simulink model "martalg1"  (Simulink 6.1)
settings: Solver=ode45  StartTime=0.0  StopTime=10.0  RelTol=1e-3
settings Model: Creator=pmosterm  LastModifiedBy=mshakeri  ExtModeAutoUpdateStatusClock=off  StrictBusMsg=ErrorLevel1
settings DataIOCC: SaveFormat=StructureWithTime  SignalLoggingName=logsOut
settings OptimizationCC: InlineParams=on  OptimizeModelRefInitCode=on  LifeSpan=1
settings ModelReferenceCC: ModelReferenceMinAlgLoopOccurrences=on
settings RTWCC: SystemTargetFile=ert.tlc  TemplateMakefile=ert_default_tmf  Description=Real-Time Workshop Embedded Coder (no auto configuration)  ProcessScript=ert_make_rtw_hook
settings CodeAppCC: IgnoreCustomStorageClasses=off  CustomSymbolStr=$N$M
settings ERTTargetCC: TargetFcnLib=ansi_tfl_tmw.mat  GenFloatMathFcnCalls=ANSI_C  GenerateSampleERTMain=on  InlinedParameterPlacement=NonHierarchical  ERTCustomFileTemplate=example_file_process.tlc  InitialValueSource=Model

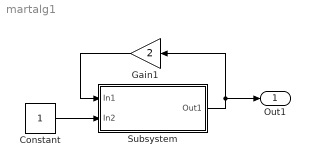
== system martalg1 ==
  Constant : Constant  SampleTime=1
  Gain1 : Gain  Orientation=left  Gain=2
  Subsystem : Subsystem  TreatAsAtomicUnit=on
      settings: MinAlgLoopOccurrences=on
  Out1 : Outport
  wires:
  Subsystem/1(Out1) -> Gain1/1, Out1/1
  Constant/1 -> Subsystem/2(In2)
  Gain1/1 -> Subsystem/1(In1)

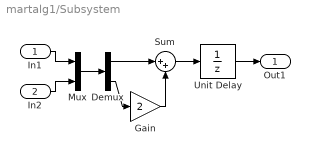
== system martalg1/Subsystem ==
  In1 : Inport  Port=1  LatchInput=off
  In2 : Inport  Port=2  LatchInput=off
  Demux : Demux  Outputs=2
  Gain : Gain  Gain=2
  Mux : Mux  Inputs=2
  Sum : Sum  Inputs=|++
  Unit Delay : UnitDelay
  Out1 : Outport
  wires:
  Sum/1 -> Unit Delay/1
  Demux/1 -> Sum/1
  Gain/1 -> Sum/2
  Demux/2 -> Gain/1
  Mux/1 -> Demux/1
  In1/1 -> Mux/1
  Unit Delay/1 -> Out1/1
  In2/1 -> Mux/2
